simulink model "sf_superstep"  (R2015b)
settings: Solver=FixedStepDiscrete  SolverMode=SingleTasking  StartTime=0.0  StopTime=40/100  RelTol=1e-3
settings Model: Creator=at-mt  LastModifiedBy=amatsumo
settings DataIOCC: SaveFormat=Array  SignalLoggingSaveFormat=ModelDataLogs  SaveOutput=off  SignalLogging=off  SaveTime=off
settings OptimizationCC: BlockReduction=off  ConditionallyExecuteInputs=off  DefaultParameterBehavior=Inlined  ExpressionDepthLimit=2147483647
settings DebuggingCC: AlgebraicLoopMsg=error  UnderspecifiedInitializationDetection=Classic  MergeDetectMultiDrivingBlocksExec=none  SolverPrmCheckMsg=warning  SingleTaskRateTransMsg=error  FcnCallInpInsideContextMsg=UseLocalSettings  StateNameClashWarn=warning
settings HardwareCC: ProdBitPerPointer=32  ProdLargestAtomicFloat=None  ProdIntDivRoundTo=Undefined  ProdEndianess=Unspecified  ProdWordSize=32  ProdHWDeviceType=ASIC/FPGA->ASIC/FPGA  ProdEqTarget=off
settings GRTTargetCC: GeneratePreprocessorConditionals=Disable all  CombineOutputUpdateFcns=off  GRTInterface=on
settings ConfigComp: CovModelRefEnable=Off  CovSFcnEnable=off

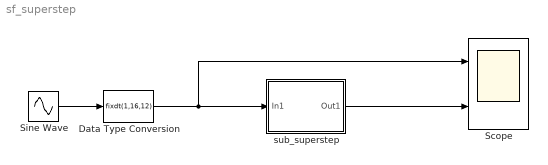
== system sf_superstep ==
  Data Type Conversion : DataTypeConversion  OutDataTypeStr=fixdt(1,16,12)
  Scope : Scope  NumInputPorts=2
  Sine Wave : Sin  Amplitude=4  Bias=0.4  Frequency=10  SampleTime=1/100
  sub_superstep : Subsystem
  wires:
  Sine Wave/1 -> Data Type Conversion/1
  Data Type Conversion/1 -> sub_superstep/1(In1), Scope/1
  sub_superstep/1(Out1) -> Scope/2

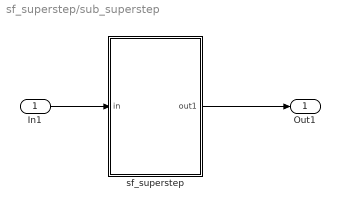
== system sf_superstep/sub_superstep ==
  In1 : Inport
  sf_superstep : Stateflow chart  TreatAsAtomicUnit=on
  Out1 : Outport
  wires:
  sf_superstep/1(out1) -> Out1/1
  In1/1 -> sf_superstep/1(in)

== stateflow chart sf_superstep/sub_superstep/sf_superstep ==
  settings: updateMethod=DISCRETE  stateMachineType=MEALY_MACHINE  executeAtInitialization=1  initializeOutput=1  enableNonTerminalStates=1
  state Init/
  state On1/
  state Off1/
  Init -> Off1 [order 2] : [in >= 0]
      | {out1 = 0;}
  (default) -> Init : {out1=10;}
  Init -> On1 [order 1] : [in < 0]
      | {out1 = 1;}
  Off1 -> Init : [in < 0]
      | {out1 = 3;}
  On1 -> Off1 : [in < 0]
      | {out1 = 2;}
  data: in input fixdt(1,16,12) size=1; out1 output int16 size=1
